simulink model "quadsim"  (R2017a)
settings: Solver=ode45  StartTime=0.0  StopTime=20  FixedStep=0.001  RelTol=1e-3  EnableMultiTasking=on
InitFcn:
  | param
undefined symbols (not defined in the file or in its folder): controller, drawAircraft, P, plotter, trajectory
settings Model: NumberOfSteps=100  Creator=ecestudent  LastModifiedBy=plusk01
settings DataIOCC: LimitDataPoints=on  SaveFormat=Array
settings OptimizationCC: LifeSpan=inf
settings DebuggingCC: SFUnexpectedBacktrackingDiag=warning  SFNoUnconditionalDefaultTransitionDiag=warning  SFExecutionAtInitializationDiag=none
settings HardwareCC: ProdBitPerPointer=32  ProdBitPerSizeT=32  ProdBitPerPtrDiffT=32  ProdLargestAtomicFloat=None  ProdIntDivRoundTo=Undefined  ProdEndianess=Unspecified  ProdWordSize=32  ProdHWDeviceType=32-bit Generic
settings ModelReferenceCC: PropagateSignalLabelsOutOfModel=off
settings GRTTargetCC: TargetLangStandard=C89/C90 (ANSI)  GeneratePreprocessorConditionals=Disable all
settings ConfigComp: CovMetricSettings=dw  CovHtmlReporting=on  CovSaveCumulativeToWorkspaceVar=on  CovSaveSingleToWorkspaceVar=on  CovExternalEMLEnable=off

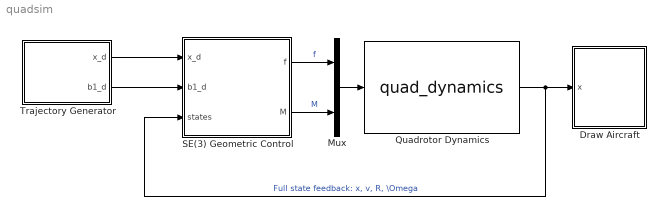
== system quadsim ==
  Draw Aircraft : Subsystem
      mask Display: image(imread('images/tv.jpg'))
  Mux : Mux  Inputs=2
  Quadrotor Dynamics : S-Function  FunctionName=quad_dynamics  Parameters=P  SFunctionDeploymentMode=off  EnableBusSupport=off
      mask Display: image(imread('images/hexacopter.png'))
  SE(3) Geometric Control : Subsystem
      mask Display: image(imread('images/boyssurface.png'))
  Trajectory Generator : Subsystem
  wires:
  Mux/1 -> Quadrotor Dynamics/1
  Quadrotor Dynamics/1 -> Draw Aircraft/1(x), SE(3) Geometric Control/3(states)  "Full state feedback: x, v, R, \\Omega"
  SE(3) Geometric Control/1(f) -> Mux/1  "f"
  SE(3) Geometric Control/2(M) -> Mux/2  "M"
  Trajectory Generator/1(x_d) -> SE(3) Geometric Control/1(x_d)
  Trajectory Generator/2(b1_d) -> SE(3) Geometric Control/2(b1_d)

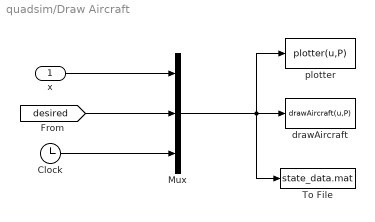
== system quadsim/Draw Aircraft ==
  x : Inport
  Clock : Clock
  Mux : Mux  Inputs=3
  To File : ToFile  Filename=state_data.mat  MatrixName=state_data
  drawAircraft : MATLABFcn  MATLABFcn=drawAircraft(u,P)  OutputDimensions=0  SampleTime=0.05
  plotter : MATLABFcn  MATLABFcn=plotter(u,P)  OutputDimensions=0  SampleTime=0.05
  wires:
  x/1 -> Mux/1
  [desired] -> Mux/2
  Mux/1 -> To File/1, plotter/1, drawAircraft/1
  Clock/1 -> Mux/3

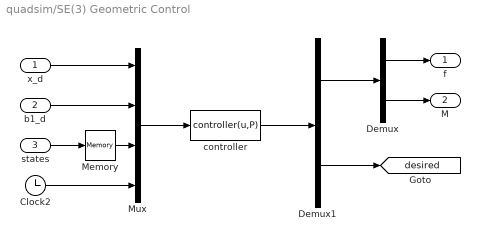
== system quadsim/SE(3) Geometric Control ==
  x_d : Inport
  b1_d : Inport  Port=2
  states : Inport  Port=3
  Clock2 : Clock
  Demux : Demux  Outputs=2
  Demux1 : Demux  Outputs=[4;6]
  Memory : Memory
  Mux : Mux
  controller : MATLABFcn  MATLABFcn=controller(u,P)  OutputDimensions=10  SampleTime=P.Ts
  f : Outport
  M : Outport  Port=2
  tag scope: desired=global
  wires:
  Clock2/1 -> Mux/4
  Mux/1 -> controller/1
  states/1 -> Memory/1
  x_d/1 -> Mux/1
  Memory/1 -> Mux/3
  controller/1 -> Demux1/1
  Demux/1 -> f/1
  Demux/2 -> M/1
  b1_d/1 -> Mux/2
  Demux1/1 -> Demux/1
  Demux1/2 -> [desired]

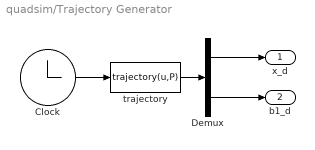
== system quadsim/Trajectory Generator ==
  Clock : Clock
  Demux : Demux  Outputs=2
  trajectory : MATLABFcn  MATLABFcn=trajectory(u,P)  OutputDimensions=6
  x_d : Outport
  b1_d : Outport  Port=2
  wires:
  Clock/1 -> trajectory/1
  trajectory/1 -> Demux/1
  Demux/1 -> x_d/1
  Demux/2 -> b1_d/1
